simulink model "Tidal_model_1"  (R2018a)
settings: Solver=VariableStepAuto  StartTime=0.0  StopTime=10.0  RelTol=1e-3
settings Model: Creator=DELL  LastModifiedBy=DELL

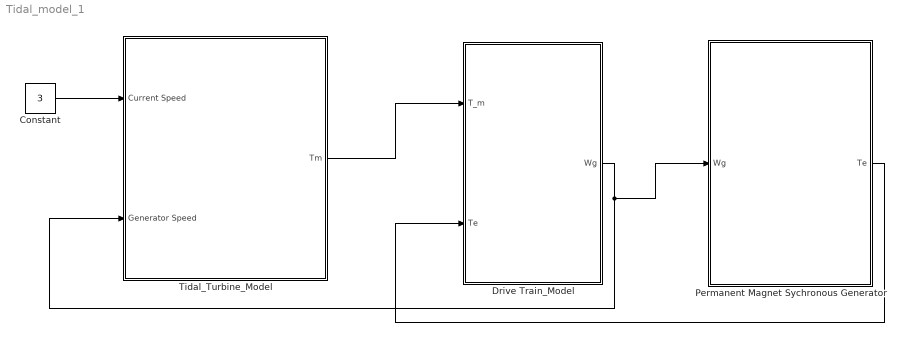
== system Tidal_model_1 ==
  Constant : Constant  Value=3
  Drive Train_Model : Subsystem
  Permanent Magnet Sychronous Generator : Subsystem
  Tidal_Turbine_Model : Subsystem
  wires:
  Constant/1 -> Tidal_Turbine_Model/1(Current Speed)
  Drive Train_Model/1(Wg) -> Permanent Magnet Sychronous Generator/1(Wg), Tidal_Turbine_Model/2(Generator Speed)
  Tidal_Turbine_Model/1(Tm) -> Drive Train_Model/1(T_m)
  Permanent Magnet Sychronous Generator/1(Te) -> Drive Train_Model/2(Te)

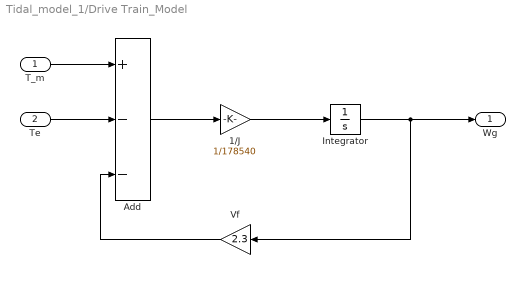
== system Tidal_model_1/Drive Train_Model ==
  T_m : Inport
  Te : Inport  Port=2
  1/J : Gain  Gain=1/178540
  Add : Sum  Inputs=+--
  Integrator : Integrator
  Vf : Gain  Gain=2.3
  Wg : Outport
  wires:
  Vf/1 -> Add/3
  T_m/1 -> Add/1
  Integrator/1 -> Wg/1, Vf/1
  Te/1 -> Add/2
  Add/1 -> 1/J/1
  1/J/1 -> Integrator/1

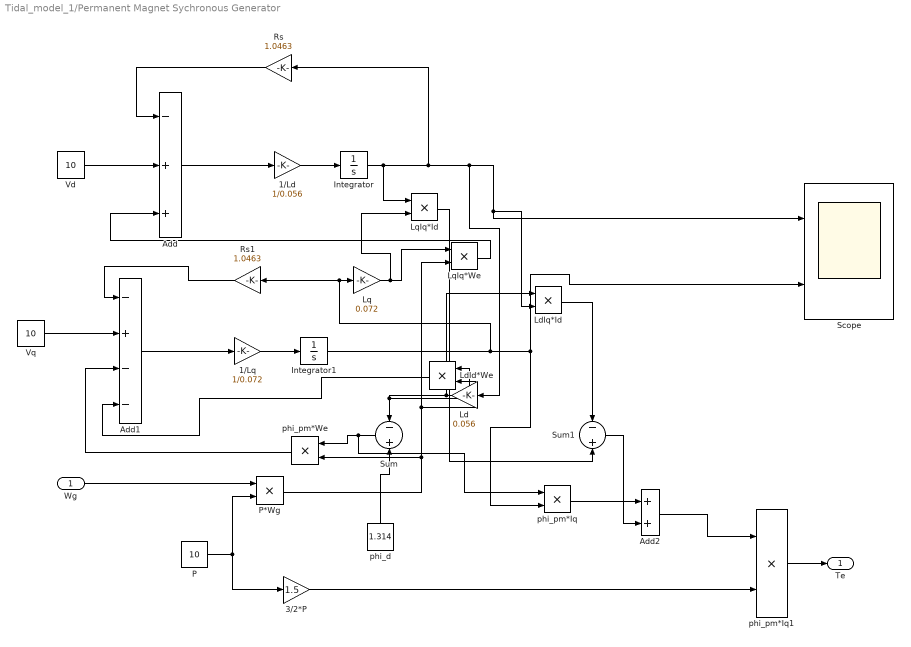
== system Tidal_model_1/Permanent Magnet Sychronous Generator ==
  Wg : Inport
  1/Ld : Gain  Gain=1/0.056
  1/Lq : Gain  Gain=1/0.072
  3/2*P : Gain  Gain=1.5
  Add : Sum  Inputs=-++
  Add1 : Sum  Inputs=-+--
  Add2 : Sum
  Integrator : Integrator
  Integrator1 : Integrator
  Ld : Gain  Gain=0.056
  LdId*We : Product
  LdIq*Id : Product
  Lq : Gain  Gain=0.072
  LqIq*Id : Product
  LqIq*We : Product
  P : Constant  Value=10
  P*Wg : Product
  Rs : Gain  Gain=1.0463
  Rs1 : Gain  Gain=1.0463
  Scope : Scope  NumInputPorts=2
  Sum : Sum  Inputs=-+
  Sum1 : Sum  Inputs=-+
  Vd : Constant  Value=10
  Vq : Constant  Value=10
  phi_d : Constant  Value=1.314
  phi_pm*Iq : Product
  phi_pm*Iq1 : Product
  phi_pm*We : Product
  Te : Outport
  wires:
  P/1 -> 3/2*P/1, P*Wg/2
  P*Wg/1 -> phi_pm*We/2, LdId*We/2, LqIq*We/2
  1/Ld/1 -> Integrator/1
  Wg/1 -> P*Wg/1
  Vd/1 -> Add/2
  Add/1 -> 1/Ld/1
  Integrator/1 -> LqIq*Id/1, Rs/1, Ld/1, Scope/1, LdIq*Id/2
  LdId*We/1 -> Add1/4
  1/Lq/1 -> Integrator1/1
  Add1/1 -> 1/Lq/1
  Lq/1 -> LqIq*Id/2, LqIq*We/1
  Integrator1/1 -> Rs1/1, Lq/1, Scope/2, phi_pm*Iq/2
  LqIq*We/1 -> Add/3
  Rs/1 -> Add/1
  Ld/1 -> LdIq*Id/1, LdId*We/1, Sum/1
  Rs1/1 -> Add1/1
  Vq/1 -> Add1/2
  Sum/1 -> phi_pm*Iq/1, phi_pm*We/1
  phi_d/1 -> Sum/2
  phi_pm*We/1 -> Add1/3
  LqIq*Id/1 -> Sum1/2
  LdIq*Id/1 -> Sum1/1
  phi_pm*Iq/1 -> Add2/1
  Sum1/1 -> Add2/2
  Add2/1 -> phi_pm*Iq1/1
  3/2*P/1 -> phi_pm*Iq1/2
  phi_pm*Iq1/1 -> Te/1

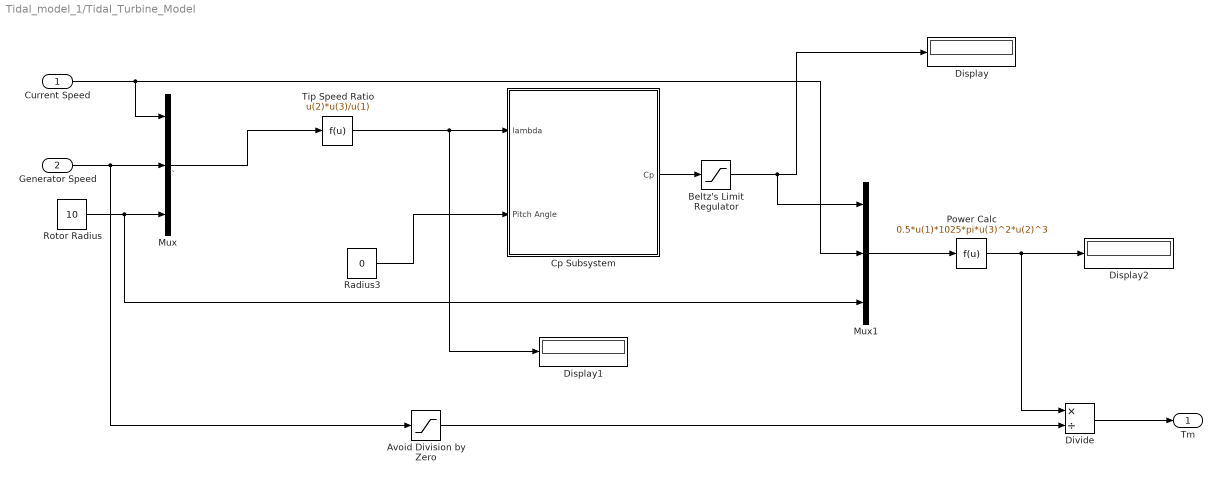
== system Tidal_model_1/Tidal_Turbine_Model ==
  note: `
  Current Speed : Inport
  Generator Speed : Inport  Port=2
  Avoid Division by Zero : Saturate  UpperLimit=inf  LowerLimit=1e-6
  Beltz's Limit Regulator : Saturate  UpperLimit=0.592  LowerLimit=1e-6
  Cp Subsystem : Subsystem
  Display : Display
  Display1 : Display
  Display2 : Display
  Divide : Product  Inputs=*/
  Mux : Mux  Inputs=3
  Mux1 : Mux  Inputs=3
  Power Calc : Fcn  Expr=0.5*u(1)*1025*pi*u(3)^2*u(2)^3
  Radius3 : Constant  Value=0
  Rotor Radius : Constant  Value=10
  "Tip Speed Ratio " : Fcn  Expr=u(2)*u(3)/u(1)
  Tm : Outport
  wires:
  Rotor Radius/1 -> Mux1/3, Mux/3
  Power Calc/1 -> Divide/1, Display2/1
  Mux1/1 -> Power Calc/1
  Divide/1 -> Tm/1
  "Tip Speed Ratio "/1 -> Display1/1, Cp Subsystem/1(lambda)
  Avoid Division by Zero/1 -> Divide/2
  Generator Speed/1 -> Avoid Division by Zero/1, Mux/2
  Mux/1 -> "Tip Speed Ratio "/1
  Beltz's Limit Regulator/1 -> Mux1/1, Display/1
  Radius3/1 -> Cp Subsystem/2(Pitch Angle)
  Cp Subsystem/1(Cp) -> Beltz's Limit Regulator/1
  Current Speed/1 -> Mux/1, Mux1/2

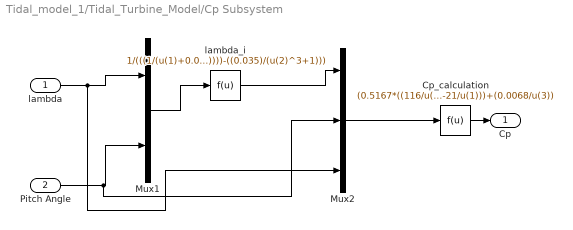
== system Tidal_model_1/Tidal_Turbine_Model/Cp Subsystem ==
  lambda : Inport
  Pitch Angle : Inport  Port=2
  Cp_calculation : Fcn  Expr=(0.5167*((116/u(1)) - (0.4*u(2)) - (5))*exp(-21/u(1)))+(0.0068/u(3))
  Mux1 : Mux  Inputs=2
  Mux2 : Mux  Inputs=3
  lambda_i : Fcn  Expr=1/(((1/(u(1)+0.08*u(2))))-((0.035)/(u(2)^3+1)))
  Cp : Outport
  wires:
  Pitch Angle/1 -> Mux2/2, Mux1/2
  Mux1/1 -> lambda_i/1
  Mux2/1 -> Cp_calculation/1
  lambda/1 -> Mux2/3, Mux1/1
  Cp_calculation/1 -> Cp/1
  lambda_i/1 -> Mux2/1
